simulink model "simulink_to_apollo_2015a_v2"  (R2015a)
settings: Solver=ode45  SolverMode=SingleTasking  StartTime=0.0  StopTime=inf  RelTol=1e-3
model workspace (MAT data in the model file):
  SL_ROS_VariableLengthArrays_MaxSizes.CommonInfo.ArrayTruncateAction = 'EmitWarning'
  SL_ROS_VariableLengthArrays_MaxSizes.MsgTypeMap = containers.Map
  SL_ROS_VariableLengthArrays_MaxSizes.MsgTypeMap.serialization.keys = {'my_msgs/ContiRadar', 'my_msgs/Header', 'my_msgs/RoutingRequest', 'sensor_msgs/PointCloud2'}
  SL_ROS_VariableLengthArrays_MaxSizes.MsgTypeMap.serialization.values{1}.PropertyName = 'Contiobs'
  SL_ROS_VariableLengthArrays_MaxSizes.MsgTypeMap.serialization.values{1}.DataType = 'my_msgs/ContiRadarObs'
  SL_ROS_VariableLengthArrays_MaxSizes.MsgTypeMap.serialization.values{1}.MaxLength = 9
  SL_ROS_VariableLengthArrays_MaxSizes.MsgTypeMap.serialization.values{2}.PropertyName = 'ModuleName'
  SL_ROS_VariableLengthArrays_MaxSizes.MsgTypeMap.serialization.values{2}.DataType = 'uint8'
  SL_ROS_VariableLengthArrays_MaxSizes.MsgTypeMap.serialization.values{2}.MaxLength = 1
  SL_ROS_VariableLengthArrays_MaxSizes.MsgTypeMap.serialization.values{3}(1).PropertyName = 'BlacklistedRoad'
  SL_ROS_VariableLengthArrays_MaxSizes.MsgTypeMap.serialization.values{3}(1).DataType = 'std_msgs/String'
  SL_ROS_VariableLengthArrays_MaxSizes.MsgTypeMap.serialization.values{3}(1).MaxLength = 16
  SL_ROS_VariableLengthArrays_MaxSizes.MsgTypeMap.serialization.values{3}(2).PropertyName = 'Waypoint'
  SL_ROS_VariableLengthArrays_MaxSizes.MsgTypeMap.serialization.values{3}(2).DataType = 'my_msgs/LaneWayPoint'
  SL_ROS_VariableLengthArrays_MaxSizes.MsgTypeMap.serialization.values{3}(2).MaxLength = 2
  SL_ROS_VariableLengthArrays_MaxSizes.MsgTypeMap.serialization.values{4}(1).PropertyName = 'Data'
  SL_ROS_VariableLengthArrays_MaxSizes.MsgTypeMap.serialization.values{4}(1).DataType = 'uint8'
  SL_ROS_VariableLengthArrays_MaxSizes.MsgTypeMap.serialization.values{4}(1).MaxLength = 128
  SL_ROS_VariableLengthArrays_MaxSizes.MsgTypeMap.serialization.values{4}(2).PropertyName = 'Fields'
  SL_ROS_VariableLengthArrays_MaxSizes.MsgTypeMap.serialization.values{4}(2).DataType = 'sensor_msgs/PointField'
  SL_ROS_VariableLengthArrays_MaxSizes.MsgTypeMap.serialization.values{4}(2).MaxLength = 4
  SL_ROS_VariableLengthArrays_MaxSizes.MsgTypeMap.serialization.uniformity = 0
  SL_ROS_VariableLengthArrays_MaxSizes.MsgTypeMap.serialization.keyType = 'char'
  SL_ROS_VariableLengthArrays_MaxSizes.MsgTypeMap.serialization.valueType = 'any'
undefined symbols (not defined in the file): CameraTimestamp, Confidence, ConfidenceType, Contiobs, Contiobs_SL_Info, Count, Data, Datatype, ErrorCode, Fields, Fields_SL_Info, Header, Height, Id, Id_SL_Info, Imu, Length, LidarTimestamp, Name, Name_SL_Info, ObjectListStatus, Offset, PerceptionObstacle, PerceptionObstacle_SL_Info, PointStep, PolygonPoint, PolygonPoint_SL_Info, Pose, Position, RadarTimestamp, RowStep, S, SequenceNum, Theta, Timestamp, TimestampSec, TrackingTime, Type, Velocity, Waypoint, Width, X, Y, Z
libraries: robotlib x35
settings Model: CovMetricSettings=dwe  CovHtmlReporting=off  covSaveCumulativeToWorkspaceVar=off  CovSaveSingleToWorkspaceVar=off  CovExternalEMLEnable=on  Creator=mskim  LastModifiedBy=mskim
settings DataIOCC: LimitDataPoints=off  SaveFormat=Dataset
settings DebuggingCC: SFUnexpectedBacktrackingDiag=error  SFNoUnconditionalDefaultTransitionDiag=error
settings HardwareCC: ProdBitPerPointer=64  ProdLargestAtomicFloat=Float  ProdIntDivRoundTo=Zero  ProdEndianess=LittleEndian  ProdHWDeviceType=Specified
settings ModelReferenceCC: PropagateSignalLabelsOutOfModel=on
settings SFSimCC: SimUseLocalCustomCode=on
settings RTWCC: RTWUseLocalCustomCode=on
settings GRTTargetCC: TargetLangStandard=C99 (ISO)  GeneratePreprocessorConditionals=Use local settings

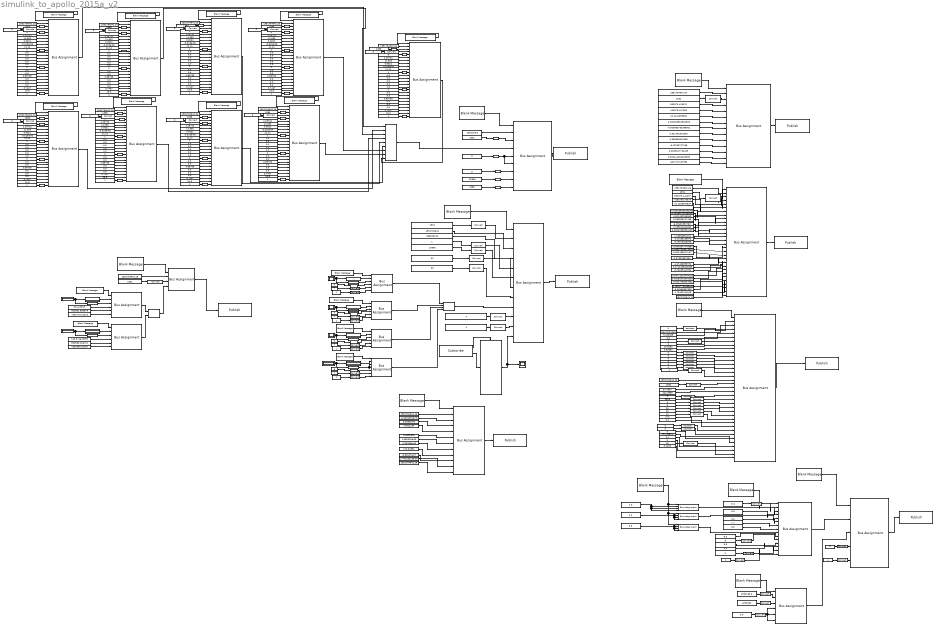
== system simulink_to_apollo_2015a_v2 ==
  note: 32
  note: 6
  note: 30
  note: 0
  note: 26
  note: 24
  note: 17
  note: 11
  Blank Message : robotlib/Blank Message  messageClass=Message  entityType=my_msgs/Gps  messageType=my_msgs/Gps  SampleTime=inf
  Blank Message1 : robotlib/Blank Message  messageClass=Message  entityType=my_msgs/LocalizationEstimate  messageType=my_msgs/LocalizationEstimate  SampleTime=inf
  Blank Message{10..18} (9 alike) : robotlib/Blank Message  messageClass=Message  entityType=my_msgs/ContiRadarObs  messageType=my_msgs/ContiRadarObs  SampleTime=inf
  Blank Message19 : robotlib/Blank Message  messageClass=Message  entityType=my_msgs/RoutingRequest  messageType=my_msgs/RoutingRequest  SampleTime=inf
  Blank Message2 : robotlib/Blank Message  messageClass=Message  entityType=my_msgs/CorrectedImu  messageType=my_msgs/CorrectedImu  SampleTime=inf
  Blank Message20 : robotlib/Blank Message  messageClass=Message  entityType=my_msgs/LaneWayPoint  messageType=my_msgs/LaneWayPoint  SampleTime=inf
  Blank Message21 : robotlib/Blank Message  messageClass=Message  entityType=my_msgs/LaneWayPoint  messageType=my_msgs/LaneWayPoint  SampleTime=inf
  Blank Message22 : robotlib/Blank Message  messageClass=Message  entityType=my_msgs/Header  messageType=my_msgs/Header  SampleTime=inf
  Blank Message23 : robotlib/Blank Message  messageClass=Message  entityType=my_msgs/PerceptionObstacle  messageType=my_msgs/PerceptionObstacle  SampleTime=inf
  Blank Message24 : robotlib/Blank Message  messageClass=Message  entityType=my_msgs/Point3D  messageType=my_msgs/Point3D  SampleTime=inf
  Blank Message25 : robotlib/Blank Message  messageClass=Message  entityType=my_msgs/PerceptionObstacles  messageType=my_msgs/PerceptionObstacles  SampleTime=inf
  Blank Message3 : robotlib/Blank Message  messageClass=Message  entityType=sensor_msgs/PointCloud2  messageType=sensor_msgs/PointCloud2  SampleTime=inf
  Blank Message{4..6,8} (4 alike) : robotlib/Blank Message  messageClass=Message  entityType=sensor_msgs/PointField  messageType=sensor_msgs/PointField  SampleTime=inf
  Blank Message7 : robotlib/Blank Message  messageClass=Message  entityType=my_msgs/Chassis  messageType=my_msgs/Chassis  SampleTime=inf
  Blank Message9 : robotlib/Blank Message  messageClass=Message  entityType=my_msgs/ContiRadar  messageType=my_msgs/ContiRadar  SampleTime=inf
  Bus Assignment : BusAssignment  AssignedSignals=Header.TimestampSec,Header.SequenceNum,Localization.Position.X,Localization.Position.Y,Localization.Position.Z,Localization.Orientation.Qx,Localization.Orientation.Qy,Localization.Orientation.Qz,Localization.Orientation.Qw,Localization.LinearVelocity.X,Localization.LinearVelocity.Y,Localization.LinearVelocity.Z,Localization.Heading
  Bus Assignment1 : BusAssignment  AssignedSignals=Header.TimestampSec,Header.SequenceNum,Pose.Position.X,Pose.Position.Y,Pose.Position.Z,Pose.Orientation.Qx,Pose.Orientation.Qy,Pose.Orientation.Qz,Pose.Orientation.Qw,Pose.LinearVelocity.X,Pose.LinearVelocity.Y,Pose.LinearVelocity.Z,Pose.LinearAccelration.X,Pose.LinearAccelration.Y,Pose.LinearAccelration.Z,Pose.AngularVelocity.X,Pose.AngularVelocity.Y,Pose.AngularVelocity.Z,Pose.Heading,Pose.LinearAccelerationVrf.X,Pose.LinearAccelerationVrf.Y,Pose.LinearAccelerationVrf.Z,Pose.AngularAccelerationVrf.X,Pose.AngularAccelerationVrf.Y,Pose.AngularAccelerationVrf.Z,Pose.EulerAngles.X,Pose.EulerAngles.Y,Pose.EulerAngles.Z,MeasurementTime
  Bus Assignment{10..18} (9 alike) : BusAssignment  AssignedSignals=Header.TimestampSec,Header.SequenceNum,Clusterortrack,ObstacleId,LongitudeDist,LateralDist,LongitudeVel,LateralVel,Rcs,Dynprop,LongitudeDistRms,LateralDistRms,LongitudeVelRms,LateralVelRms,Probexist,MeasState,LongitudeAccel,LateralAccel,OritationAngle,LongitudeAccelRms,LateralAccelRms,OritationAngleRms,Length,Width,ObstacleClass
  Bus Assignment19 : BusAssignment  AssignedSignals=Header.TimestampSec,Header.SequenceNum,Waypoint
  Bus Assignment2 : BusAssignment  AssignedSignals=Header.TimestampSec,Imu.LinearAccelration.X,Imu.LinearAccelration.Y,Imu.LinearAccelration.Z,Imu.AngularVelocity.X,Imu.AngularVelocity.Y,Imu.AngularVelocity.Z,Imu.Heading,Imu.EulerAngles.X,Imu.EulerAngles.Y,Imu.EulerAngles.Z
  Bus Assignment20 : BusAssignment  AssignedSignals=Id,Id_SL_Info.CurrentLength,S,Pose.X,Pose.Y
  Bus Assignment21 : BusAssignment  AssignedSignals=Id,Id_SL_Info.CurrentLength,S,Pose.X,Pose.Y
  Bus Assignment22 : BusAssignment  AssignedSignals=TimestampSec,SequenceNum,LidarTimestamp,CameraTimestamp,RadarTimestamp
  Bus Assignment23 : BusAssignment  AssignedSignals=Id,Position,Theta,Velocity,Length,Width,Height,PolygonPoint,TrackingTime,Type,Timestamp,Confidence,ConfidenceType,PolygonPoint_SL_Info.CurrentLength
  Bus Assignment24 : BusAssignment  AssignedSignals=X,Y,Z
  Bus Assignment25 : BusAssignment  AssignedSignals=X,Y,Z
  Bus Assignment26 : BusAssignment  AssignedSignals=X,Y,Z
  Bus Assignment27 : BusAssignment  AssignedSignals=PerceptionObstacle,Header,ErrorCode,PerceptionObstacle_SL_Info.CurrentLength
  Bus Assignment3 : BusAssignment  AssignedSignals=Header.Seq,Header.Stamp.Sec,Header.Stamp.Nsec,Height,Width,PointStep,RowStep,Fields,Fields_SL_Info.CurrentLength,Fields_SL_Info.ReceivedLength,Data
  Bus Assignment4 : BusAssignment  AssignedSignals=Name,Name_SL_Info.CurrentLength,Offset,Datatype,Count
  Bus Assignment5 : BusAssignment  AssignedSignals=Name,Name_SL_Info.CurrentLength,Offset,Datatype,Count
  Bus Assignment6 : BusAssignment  AssignedSignals=Name,Name_SL_Info.CurrentLength,Offset,Datatype,Count
  Bus Assignment7 : BusAssignment  AssignedSignals=EngineStarted,EngineRpm,SpeedMps,OdometerM,FuelRangeM,ThrottlePercentage,BrakePercentage,SteeringPercentage,ParkingBrake,HighBeamSignal,LowBeamSignal,LeftTurnSignal,RightTurnSignal,Wiper,DrivingMode,Header.TimestampSec,Header.SequenceNum,ChassisGps.Latitude,ChassisGps.Longitude,ChassisGps.GpsValid,ChassisGps.Year,ChassisGps.Month,ChassisGps.Day,ChassisGps.Hours,ChassisGps.Minutes,ChassisGps.Seconds,ChassisGps.CompassDirection,ChassisGps.Pdop,ChassisGps.IsGpsFault,ChassisGps.IsInferred,ChassisGps.Altitude,ChassisGps.Heading,ChassisGps.Hdop,ChassisGps.Vdop,ChassisGps.NumSatellites,ChassisGps.GpsSpeed
  Bus Assignment8 : BusAssignment  AssignedSignals=Name,Name_SL_Info.CurrentLength,Name_SL_Info.ReceivedLength,Offset,Datatype,Count
  Bus Assignment9 : BusAssignment  AssignedSignals=Header.TimestampSec,Header.SequenceNum,Contiobs,Contiobs_SL_Info.CurrentLength,Contiobs_SL_Info.ReceivedLength,ObjectListStatus.NofObjects,ObjectListStatus.MeasCounter,ObjectListStatus.InterfaceVersion
  Cast To Boolean{,1..9} (10 alike) : DataTypeConversion  OutDataTypeStr=boolean
  Constant{,13,81,99,110,116,141,166,191,216,241,266,291,316,341} (15 alike) : Constant  Value=1551784842.26
  Constant{1,14,44,82,111,342} (6 alike) : Constant  Value=1531
  Constant10 : Constant  Value=0.0829047784209
  Constant100 : Constant  Value=-0.0001554879
  Constant101 : Constant  Value=9.3063e-05
  Constant102 : Constant  Value=-9.811154
  Constant103 : Constant  Value=0.0001616
  Constant104 : Constant  Value=2.995926e-06
  Constant105 : Constant  Value=-2.82969e-09
  Constant106 : Constant  Value=270.84991
  Constant107 : Constant  Value=1532165.6
  Constant108 : Constant  Value=-5.81627e-07
  Constant109 : Constant  Value=2.44229215e-05
  Constant11 : Constant  Value=0.000244081020355
  Constant112 : Constant  Value=9
  Constant113 : Constant  Value=9
  Constant114 : Constant  Value=22800
  Constant115 : Constant  Value=1386
  Constant{117,142,167,192,217,242,267,292,317} (9 alike) : Constant  Value=1385
  Constant{118,143,168,193,218,243,268,293,318} (9 alike) : Constant  Value=2.25722
  Constant{42..43,45..46,55..57,63,70..71,91..92,98,119,144,169,194,219,244,269..270,294,319,352} (24 alike) : Constant  Value=0
  Constant12 : Constant  Value=-225.727157593
  Constant120 : Constant  Value=6
  Constant{121,146,171,196,221,246,271,296,321} (9 alike) : Constant  Value=11.933
  Constant{122,147,172,197,222,247,272,297,322} (9 alike) : Constant  Value=-3.619e-06
  Constant{123,148,173,198,223,248,273,298,323} (9 alike) : Constant  Value=0.0021
  Constant{124,149,174,199,224,249,274,299,324} (9 alike) : Constant  Value=11.11
  Constant{69,125,127..129,131,133..134,136,138,150,152..154,156,158..159,161,163,175,177..179,181,183..184,186,188,200,202..204,206,208..209,211,213,225,227..229,231,233..234,236,238,250,252..254,256,258..259,261,263,275,277..279,281,283..284,286,288,300,302..304,306,308..309,311,313,325,327..329,331,333..334,336,338,361} (83 alike) : Constant  Value=0.0
  Constant{49,53,65..66,76,79..80,126,140,151,165,176,190,201,215,226,240,251,265,276,290,295,301,315,326,340,357..359} (29 alike) : Constant
  Constant{130,155,180,205,230,255,280,305,330,364} (10 alike) : Constant  Value=1.0
  Constant{95,132,157,182,207,220,232,257,282,307,332} (11 alike) : Constant  Value=2
  Constant{135,160,185,210,235,260,285,310,335} (9 alike) : Constant  Value=0.85705
  Constant{137,162,187,212,237,262,287,312,337} (9 alike) : Constant  Value=3.7407
  Constant{139,164,189,214,239,264,289,314,339} (9 alike) : Constant  Value=10.6
  Constant{52,62,64,75,145} (5 alike) : Constant  Value=7
  Constant15 : Constant  Value=0.00012568384409
  Constant16 : Constant  Value=1.10996984434
  Constant17 : Constant  Value=-1.27253139942
  Constant{51,59..60,170} (4 alike) : Constant  Value=4
  Constant18 : Constant  Value=552873.141037
  Constant19 : Constant  Value=4182766.70679
  Constant195 : Constant  Value=5
  Constant2 : Constant  Value=552870.429222
  Constant20 : Constant  Value=10.1238040924
  Constant21 : Constant  Value=0.000253551552305
  Constant22 : Constant  Value=-0.000893782998901
  Constant23 : Constant  Value=0.921432316303
  Constant24 : Constant  Value=-6.19401931763
  Constant245 : Constant  Value=3
  Constant25 : Constant  Value=0.139211624861
  Constant26 : Constant  Value=-9.75978325506
  Constant27 : Constant  Value=-0.0043677779987
  Constant28 : Constant  Value=0.00567089976961
  Constant29 : Constant  Value=-0.0024595711077
  Constant3 : Constant  Value=4182784.07053
  Constant30 : Constant  Value=-2.37322587092
  Constant31 : Constant  Value=-1.67436599731
  Constant32 : Constant  Value=0.0740453600883
  Constant320 : Constant  Value=8
  Constant33 : Constant  Value=0.390536427498
  Constant34 : Constant  Value=-9.76195441931
  Constant343 : Constant  Value=20.412915
  Constant344 : Constant  Value=552881.650878
  Constant345 : Constant  Value=4182775.01019
  Constant346 : Constant  Value=113.374625055
  Constant347 : Constant  Value=552880.126721
  Constant348 : Constant  Value=4182806.92204
  Constant349 : Constant  Value=1532165.6
  Constant35 : Constant  Value=0.00711610494182
  Constant350 : Constant  Value=3.5
  Constant351 : Constant  Value=111
  Constant353 : Constant  Value=9.9
  Constant354 : Constant  Value=6.6
  Constant355 : Constant  Value=5
  Constant356 : Constant  Value=8.8
  Constant36 : Constant  Value=-0.000803495408036
  Constant360 : Constant  Value=4092962
  Constant362 : Constant  Value=2.2
  Constant363 : Constant  Value=5.5
  Constant365 : Constant  Value=6.6
  Constant366 : Constant  Value=7.7
  Constant367 : Constant  Value=8.8
  Constant37 : Constant  Value=-0.0024498004932
  Constant38 : Constant  Value=2.16947784683e-05
  Constant39 : Constant  Value=-6.28168967593
  Constant4 : Constant  Value=10.1241359982
  Constant40 : Constant  Value=4.73462104918
  Constant41 : Constant  Value=1551784841.11
  Constant47 : Constant  Value=1551784842
  Constant48 : Constant  Value=696618240
  Constant5 : Constant  Value=0.000253551552305
  Constant50 : Constant  Value=10966
  Constant54 : Constant  Value=32
  Constant58 : Constant  Value=99
  Constant6 : Constant  Value=-0.000893782998901
  Constant61 : Constant  Value=8
  Constant67 : Constant  Value=2536.82299805
  Constant68 : Constant  Value=5.123308
  Constant7 : Constant  Value=0.921432316303
  Constant72 : Constant  Value=18.5281
  Constant73 : Constant  Value=0.69582
  Constant74 : Constant  Value=8
  Constant77 : Constant  Value=37.7907
  Constant78 : Constant  Value=-122.3995
  Constant8 : Constant  Value=0.388538002968
  Constant83 : Constant  Value=2019
  Constant84 : Constant  Value=3
  Constant85 : Constant  Value=5
  Constant86 : Constant  Value=20
  Constant87 : Constant  Value=20
  Constant88 : Constant  Value=41
  Constant89 : Constant  Value=270
  Constant9 : Constant  Value=-5.12263727188
  Constant90 : Constant  Value=0.1
  Constant93 : Constant  Value=271.02511
  Constant94 : Constant  Value=0.1
  Constant96 : Constant  Value=15
  Constant97 : Constant  Value=5.1233
  Data Type Conversion{,1..99} (100 alike) : DataTypeConversion
  Enabled Subsystem : Subsystem
  Matrix Concatenate : Concatenate  NumInputs=4  Mode=Multidimensional array  ConcatenateDimension=2
  Matrix Concatenate1 : Concatenate  NumInputs=9  Mode=Multidimensional array  ConcatenateDimension=2
  Matrix Concatenate2 : Concatenate  Mode=Multidimensional array  ConcatenateDimension=2
  Publish1 : robotlib/Publish  topicSource=Specify your own  topic=/my_msgs/Gps  messageType=my_msgs/Gps  messageQueueLength=1
  Publish2 : robotlib/Publish  topicSource=Specify your own  topic=/my_msgs/LocalizationEstimate  messageType=my_msgs/LocalizationEstimate  messageQueueLength=1
  Publish3 : robotlib/Publish  topicSource=Specify your own  topic=/my_msgs/CorrectedImu  messageType=my_msgs/CorrectedImu  messageQueueLength=1
  Publish4 : robotlib/Publish  topicSource=Specify your own  topic=/sensor_msgs/PointCloud2  messageType=sensor_msgs/PointCloud2  messageQueueLength=1
  Publish5 : robotlib/Publish  topicSource=Specify your own  topic=/my_msgs/Chassis  messageType=my_msgs/Chassis  messageQueueLength=1
  Publish6 : robotlib/Publish  topicSource=Specify your own  topic=/my_msgs/ContiRadar  messageType=my_msgs/ContiRadar  messageQueueLength=1
  Publish7 : robotlib/Publish  topicSource=Specify your own  topic=/my_msgs/RoutingRequest  messageType=my_msgs/RoutingRequest  messageQueueLength=1
  Publish8 : robotlib/Publish  topicSource=Specify your own  topic=/my_msgs/PerceptionObstacles  messageType=my_msgs/PerceptionObstacles  messageQueueLength=1
  Scope : Scope
      settings: TimeRange=auto  MaxDataPoints=5000  SaveToWorkspace=off  SaveName=ScopeData  YMin=-31.875  YMax=286.875  SampleTime=-1
  String Constant1 : Subsystem  Description=Replaced Block  mask(Replaced Block){}
      mask help: This block has been replaced with an empty subsystem because it used functionality that is unavailable in Simulink R2015a.
      mask Display: fprintf('Replaced: %s\n','StringConstant')
  String Constant2 : Subsystem  Description=Replaced Block  mask(Replaced Block){}
      mask help: This block has been replaced with an empty subsystem because it used functionality that is unavailable in Simulink R2015a.
      mask Display: fprintf('Replaced: %s\n','StringConstant')
  String Constant3 : Subsystem  Description=Replaced Block  mask(Replaced Block){}
      mask help: This block has been replaced with an empty subsystem because it used functionality that is unavailable in Simulink R2015a.
      mask Display: fprintf('Replaced: %s\n','StringConstant')
  String Constant4 : Subsystem  Description=Replaced Block  mask(Replaced Block){}
      mask help: This block has been replaced with an empty subsystem because it used functionality that is unavailable in Simulink R2015a.
      mask Display: fprintf('Replaced: %s\n','StringConstant')
  String Constant5 : Subsystem  Description=Replaced Block  mask(Replaced Block){}
      mask help: This block has been replaced with an empty subsystem because it used functionality that is unavailable in Simulink R2015a.
      mask Display: fprintf('Replaced: %s\n','StringConstant')
  String Constant6 : Subsystem  Description=Replaced Block  mask(Replaced Block){}
      mask help: This block has been replaced with an empty subsystem because it used functionality that is unavailable in Simulink R2015a.
      mask Display: fprintf('Replaced: %s\n','StringConstant')
  String Length1 : Subsystem  Description=Replaced Block  mask(Replaced Block){}
      mask help: This block has been replaced with an empty subsystem because it used functionality that is unavailable in Simulink R2015a.
      mask Display: fprintf('Replaced: %s\n','StringLength')
  String Length2 : Subsystem  Description=Replaced Block  mask(Replaced Block){}
      mask help: This block has been replaced with an empty subsystem because it used functionality that is unavailable in Simulink R2015a.
      mask Display: fprintf('Replaced: %s\n','StringLength')
  String Length3 : Subsystem  Description=Replaced Block  mask(Replaced Block){}
      mask help: This block has been replaced with an empty subsystem because it used functionality that is unavailable in Simulink R2015a.
      mask Display: fprintf('Replaced: %s\n','StringLength')
  String Length4 : Subsystem  Description=Replaced Block  mask(Replaced Block){}
      mask help: This block has been replaced with an empty subsystem because it used functionality that is unavailable in Simulink R2015a.
      mask Display: fprintf('Replaced: %s\n','StringLength')
  String Length5 : Subsystem  Description=Replaced Block  mask(Replaced Block){}
      mask help: This block has been replaced with an empty subsystem because it used functionality that is unavailable in Simulink R2015a.
      mask Display: fprintf('Replaced: %s\n','StringLength')
  String Length6 : Subsystem  Description=Replaced Block  mask(Replaced Block){}
      mask help: This block has been replaced with an empty subsystem because it used functionality that is unavailable in Simulink R2015a.
      mask Display: fprintf('Replaced: %s\n','StringLength')
  String to ASCII1 : Subsystem  Description=Replaced Block  mask(Replaced Block){}
      mask help: This block has been replaced with an empty subsystem because it used functionality that is unavailable in Simulink R2015a.
      mask Display: fprintf('Replaced: %s\n','StringToASCII')
  String to ASCII2 : Subsystem  Description=Replaced Block  mask(Replaced Block){}
      mask help: This block has been replaced with an empty subsystem because it used functionality that is unavailable in Simulink R2015a.
      mask Display: fprintf('Replaced: %s\n','StringToASCII')
  String to ASCII3 : Subsystem  Description=Replaced Block  mask(Replaced Block){}
      mask help: This block has been replaced with an empty subsystem because it used functionality that is unavailable in Simulink R2015a.
      mask Display: fprintf('Replaced: %s\n','StringToASCII')
  String to ASCII4 : Subsystem  Description=Replaced Block  mask(Replaced Block){}
      mask help: This block has been replaced with an empty subsystem because it used functionality that is unavailable in Simulink R2015a.
      mask Display: fprintf('Replaced: %s\n','StringToASCII')
  String to ASCII5 : Subsystem  Description=Replaced Block  mask(Replaced Block){}
      mask help: This block has been replaced with an empty subsystem because it used functionality that is unavailable in Simulink R2015a.
      mask Display: fprintf('Replaced: %s\n','StringToASCII')
  String to ASCII6 : Subsystem  Description=Replaced Block  mask(Replaced Block){}
      mask help: This block has been replaced with an empty subsystem because it used functionality that is unavailable in Simulink R2015a.
      mask Display: fprintf('Replaced: %s\n','StringToASCII')
  Subscribe1 : robotlib/Subscribe  topicSource=Specify your own  topic=/apollo/sensor/velodyne64/compensator/PointCloud2  messageType=sensor_msgs/PointCloud2  sampleTime=-1  messageQueueLength=51
  wires:
  Constant4/1 -> Bus Assignment/6
  Data Type Conversion/1 -> Bus Assignment/3
  Constant6/1 -> Bus Assignment/8
  Constant12/1 -> Bus Assignment/14
  Constant9/1 -> Bus Assignment/11
  Constant5/1 -> Bus Assignment/7
  Constant7/1 -> Bus Assignment/9
  Constant1/1 -> Data Type Conversion/1
  Constant2/1 -> Bus Assignment/4
  Constant3/1 -> Bus Assignment/5
  Blank Message/1 -> Bus Assignment/1
  Bus Assignment/1 -> Publish1/1
  Constant8/1 -> Bus Assignment/10
  Constant11/1 -> Bus Assignment/13
  Constant10/1 -> Bus Assignment/12
  Constant/1 -> Bus Assignment/2
  Constant13/1 -> Bus Assignment1/2
  Constant18/1 -> Bus Assignment1/4
  Constant19/1 -> Bus Assignment1/5
  Constant21/1 -> Bus Assignment1/7
  Bus Assignment1/1 -> Publish2/1
  Blank Message1/1 -> Bus Assignment1/1
  Constant14/1 -> Data Type Conversion1/1
  Data Type Conversion1/1 -> Bus Assignment1/3
  Constant20/1 -> Bus Assignment1/6
  Constant22/1 -> Bus Assignment1/8
  Constant23/1 -> Bus Assignment1/9
  Constant33/1 -> Bus Assignment1/10
  Constant24/1 -> Bus Assignment1/11
  Constant25/1 -> Bus Assignment1/12
  Constant15/1 -> Bus Assignment1/13
  Constant16/1 -> Bus Assignment1/14
  Constant17/1 -> Bus Assignment1/15
  Constant26/1 -> Bus Assignment1/16
  Constant27/1 -> Bus Assignment1/17
  Constant28/1 -> Bus Assignment1/18
  Constant29/1 -> Bus Assignment1/19
  Constant30/1 -> Bus Assignment1/20
  Constant31/1 -> Bus Assignment1/21
  Constant32/1 -> Bus Assignment1/22
  Constant34/1 -> Bus Assignment1/23
  Constant35/1 -> Bus Assignment1/24
  Constant36/1 -> Bus Assignment1/25
  Constant37/1 -> Bus Assignment1/26
  Constant38/1 -> Bus Assignment1/27
  Constant39/1 -> Bus Assignment1/28
  Constant40/1 -> Bus Assignment1/29
  Constant41/1 -> Bus Assignment1/30
  Blank Message3/1 -> Bus Assignment3/1
  Constant50/1 -> Data Type Conversion6/1
  Bus Assignment3/1 -> Publish4/1
  String Length3/1(Out1) -> Bus Assignment4/3
  Data Type Conversion8/1 -> Bus Assignment3/8
  Data Type Conversion7/1 -> Bus Assignment3/7
  Constant54/1 -> Data Type Conversion7/1
  Data Type Conversion6/1 -> Bus Assignment3/6
  Constant64/1 -> Data Type Conversion10/1
  Data Type Conversion5/1 -> Bus Assignment3/5
  Constant47/1 -> Bus Assignment3/3
  Data Type Conversion11/1 -> Bus Assignment4/6
  Data Type Conversion9/1 -> Bus Assignment4/4
  Constant63/1 -> Data Type Conversion9/1
  Blank Message4/1 -> Bus Assignment4/1
  Data Type Conversion10/1 -> Bus Assignment4/5
  String Constant3/1(Out1) -> String Length3/1(In1), String to ASCII1/1(In1)
  String to ASCII1/1(Out1) -> Bus Assignment4/2
  Constant58/1 -> Data Type Conversion8/1
  Constant44/1 -> Data Type Conversion4/1
  Constant48/1 -> Bus Assignment3/4
  Constant49/1 -> Data Type Conversion5/1
  Data Type Conversion4/1 -> Bus Assignment3/2
  Constant65/1 -> Data Type Conversion11/1
  Bus Assignment4/1 -> Matrix Concatenate/1
  Constant59/1 -> Data Type Conversion15/1
  Constant60/1 -> Data Type Conversion16/1
  Constant53/1 -> Data Type Conversion13/1
  String Constant1/1(Out1) -> String Length1/1(In1), String to ASCII2/1(In1)
  Data Type Conversion14/1 -> Bus Assignment5/4
  Constant52/1 -> Data Type Conversion12/1
  Data Type Conversion13/1 -> Bus Assignment5/6
  String Length1/1(Out1) -> Bus Assignment5/3
  String to ASCII2/1(Out1) -> Bus Assignment5/2
  Blank Message5/1 -> Bus Assignment5/1
  Constant51/1 -> Data Type Conversion14/1
  Data Type Conversion12/1 -> Bus Assignment5/5
  Constant66/1 -> Data Type Conversion18/1
  String Constant2/1(Out1) -> String Length2/1(In1), String to ASCII3/1(In1)
  Data Type Conversion19/1 -> Bus Assignment6/4
  Constant62/1 -> Data Type Conversion17/1
  Data Type Conversion18/1 -> Bus Assignment6/6
  String Length2/1(Out1) -> Bus Assignment6/3
  String to ASCII3/1(Out1) -> Bus Assignment6/2
  Blank Message6/1 -> Bus Assignment6/1
  Constant61/1 -> Data Type Conversion19/1
  Data Type Conversion17/1 -> Bus Assignment6/5
  Matrix Concatenate/1 -> Bus Assignment3/9
  Data Type Conversion15/1 -> Bus Assignment3/10
  Data Type Conversion16/1 -> Bus Assignment3/11
  Bus Assignment5/1 -> Matrix Concatenate/2
  Bus Assignment6/1 -> Matrix Concatenate/3
  Constant76/1 -> Data Type Conversion26/1
  Bus Assignment8/1 -> Matrix Concatenate/4
  String to ASCII4/1(Out1) -> Bus Assignment8/2
  Constant74/1 -> Data Type Conversion27/1
  String Constant4/1(Out1) -> String Length4/1(In1), String to ASCII4/1(In1)
  Blank Message8/1 -> Bus Assignment8/1
  String Length4/1(Out1) -> Bus Assignment8/4, Bus Assignment8/3
  Constant75/1 -> Data Type Conversion25/1
  Data Type Conversion27/1 -> Bus Assignment8/5
  Data Type Conversion25/1 -> Bus Assignment8/6
  Data Type Conversion26/1 -> Bus Assignment8/7
  Blank Message7/1 -> Bus Assignment7/1
  Bus Assignment7/1 -> Publish5/1
  Constant42/1 -> Cast To Boolean/1
  Cast To Boolean/1 -> Bus Assignment7/2
  Constant67/1 -> Bus Assignment7/3
  Constant68/1 -> Bus Assignment7/4
  Constant69/1 -> Bus Assignment7/5
  Constant70/1 -> Data Type Conversion2/1
  Constant71/1 -> Bus Assignment7/7
  Constant43/1 -> Cast To Boolean1/1
  Constant45/1 -> Cast To Boolean2/1
  Constant46/1 -> Cast To Boolean3/1
  Constant57/1 -> Cast To Boolean6/1
  Constant56/1 -> Cast To Boolean5/1
  Constant55/1 -> Cast To Boolean4/1
  Constant72/1 -> Bus Assignment7/8
  Constant73/1 -> Bus Assignment7/9
  Cast To Boolean1/1 -> Bus Assignment7/10
  Cast To Boolean2/1 -> Bus Assignment7/11
  Cast To Boolean3/1 -> Bus Assignment7/12
  Cast To Boolean4/1 -> Bus Assignment7/13
  Cast To Boolean5/1 -> Bus Assignment7/14
  Cast To Boolean6/1 -> Bus Assignment7/15
  Constant80/1 -> Data Type Conversion3/1
  Constant82/1 -> Data Type Conversion20/1
  Constant81/1 -> Bus Assignment7/17
  Constant79/1 -> Cast To Boolean7/1
  Constant91/1 -> Cast To Boolean8/1
  Constant98/1 -> Cast To Boolean9/1
  Constant83/1 -> Data Type Conversion21/1
  Constant84/1 -> Data Type Conversion22/1
  Constant85/1 -> Data Type Conversion23/1
  Constant86/1 -> Data Type Conversion24/1
  Constant87/1 -> Data Type Conversion28/1
  Constant88/1 -> Data Type Conversion29/1
  Constant96/1 -> Data Type Conversion30/1
  Data Type Conversion2/1 -> Bus Assignment7/6
  Data Type Conversion3/1 -> Bus Assignment7/16
  Data Type Conversion20/1 -> Bus Assignment7/18
  Constant77/1 -> Bus Assignment7/19
  Constant78/1 -> Bus Assignment7/20
  Cast To Boolean7/1 -> Bus Assignment7/21
  Data Type Conversion21/1 -> Bus Assignment7/22
  Data Type Conversion22/1 -> Bus Assignment7/23
  Data Type Conversion23/1 -> Bus Assignment7/24
  Data Type Conversion24/1 -> Bus Assignment7/25
  Data Type Conversion28/1 -> Bus Assignment7/26
  Data Type Conversion29/1 -> Bus Assignment7/27
  Constant89/1 -> Bus Assignment7/28
  Constant90/1 -> Bus Assignment7/29
  Cast To Boolean8/1 -> Bus Assignment7/30
  Cast To Boolean9/1 -> Bus Assignment7/31
  Constant92/1 -> Bus Assignment7/32
  Constant93/1 -> Bus Assignment7/33
  Constant94/1 -> Bus Assignment7/34
  Constant95/1 -> Bus Assignment7/35
  Data Type Conversion30/1 -> Bus Assignment7/36
  Constant97/1 -> Bus Assignment7/37
  Blank Message2/1 -> Bus Assignment2/1
  Bus Assignment2/1 -> Publish3/1
  Constant99/1 -> Bus Assignment2/2
  Constant100/1 -> Bus Assignment2/3
  Constant101/1 -> Bus Assignment2/4
  Constant102/1 -> Bus Assignment2/5
  Constant103/1 -> Bus Assignment2/6
  Constant104/1 -> Bus Assignment2/7
  Constant105/1 -> Bus Assignment2/8
  Constant106/1 -> Bus Assignment2/9
  Constant108/1 -> Bus Assignment2/10
  Constant109/1 -> Bus Assignment2/11
  Constant110/1 -> Bus Assignment2/12
  Subscribe1/2 -> Enabled Subsystem/1(In1)
  Subscribe1/1 -> Enabled Subsystem/Enable
  Enabled Subsystem/1(Out1) -> Scope/1, Bus Assignment3/12
  Blank Message9/1 -> Bus Assignment9/1
  Bus Assignment9/1 -> Publish6/1
  Constant327/1 -> Bus Assignment18/13
  Constant316/1 -> Bus Assignment18/2
  Constant339/1 -> Bus Assignment18/25
  Constant318/1 -> Bus Assignment18/6
  Constant336/1 -> Bus Assignment18/22
  Constant322/1 -> Bus Assignment18/9
  Constant330/1 -> Bus Assignment18/16
  Constant324/1 -> Bus Assignment18/10
  Constant319/1 -> Data Type Conversion39/1
  Constant334/1 -> Bus Assignment18/21
  Constant328/1 -> Bus Assignment18/15
  Constant325/1 -> Bus Assignment18/12
  Constant323/1 -> Bus Assignment18/8
  Constant333/1 -> Bus Assignment18/19
  Constant335/1 -> Bus Assignment18/20
  Data Type Conversion39/1 -> Bus Assignment18/4
  Constant338/1 -> Bus Assignment18/23
  Constant321/1 -> Bus Assignment18/7
  Constant337/1 -> Bus Assignment18/24
  Constant329/1 -> Bus Assignment18/14
  Constant331/1 -> Bus Assignment18/18
  Blank Message18/1 -> Bus Assignment18/1
  Constant317/1 -> Data Type Conversion42/1
  Data Type Conversion42/1 -> Bus Assignment18/3
  Constant340/1 -> Data Type Conversion49/1
  Data Type Conversion49/1 -> Bus Assignment18/26
  Constant332/1 -> Data Type Conversion50/1
  Data Type Conversion50/1 -> Bus Assignment18/17
  Constant326/1 -> Data Type Conversion61/1
  Data Type Conversion61/1 -> Bus Assignment18/11
  Constant320/1 -> Data Type Conversion83/1
  Data Type Conversion83/1 -> Bus Assignment18/5
  Bus Assignment18/1 -> Matrix Concatenate1/9
  Constant107/1 -> Bus Assignment9/2
  Constant111/1 -> Data Type Conversion31/1
  Data Type Conversion31/1 -> Bus Assignment9/3
  Constant112/1 -> Data Type Conversion32/1
  Data Type Conversion32/1 -> Bus Assignment9/6, Bus Assignment9/5
  Constant113/1 -> Data Type Conversion87/1
  Constant114/1 -> Data Type Conversion88/1
  Constant115/1 -> Data Type Conversion89/1
  Bus Assignment12/1 -> Matrix Concatenate1/5
  Bus Assignment14/1 -> Matrix Concatenate1/3
  Bus Assignment15/1 -> Matrix Concatenate1/4
  Bus Assignment16/1 -> Matrix Concatenate1/1
  Bus Assignment13/1 -> Matrix Concatenate1/6
  Constant287/1 -> Bus Assignment16/24
  Blank Message13/1 -> Bus Assignment13/1
  Data Type Conversion54/1 -> Bus Assignment11/26
  Data Type Conversion47/1 -> Bus Assignment15/3
  Constant188/1 -> Bus Assignment12/23
  Constant263/1 -> Bus Assignment15/23
  Data Type Conversion70/1 -> Bus Assignment14/17
  Data Type Conversion45/1 -> Bus Assignment12/3
  Constant283/1 -> Bus Assignment16/19
  Constant190/1 -> Data Type Conversion57/1
  Data Type Conversion73/1 -> Bus Assignment17/26
  Constant241/1 -> Bus Assignment15/2
  Blank Message10/1 -> Bus Assignment10/1
  Constant289/1 -> Bus Assignment16/25
  Constant119/1 -> Data Type Conversion33/1
  Constant142/1 -> Data Type Conversion44/1
  Bus Assignment11/1 -> Matrix Concatenate1/8
  Data Type Conversion56/1 -> Bus Assignment13/17
  Blank Message12/1 -> Bus Assignment12/1
  Constant181/1 -> Bus Assignment12/18
  Constant173/1 -> Bus Assignment12/8
  Constant202/1 -> Bus Assignment13/13
  Data Type Conversion74/1 -> Bus Assignment17/17
  Constant194/1 -> Data Type Conversion36/1
  Constant245/1 -> Data Type Conversion86/1
  Blank Message14/1 -> Bus Assignment14/1
  Data Type Conversion57/1 -> Bus Assignment12/26
  Constant133/1 -> Bus Assignment10/19
  Constant199/1 -> Bus Assignment13/10
  Constant205/1 -> Bus Assignment13/16
  Constant152/1 -> Bus Assignment11/13
  Constant209/1 -> Bus Assignment13/21
  Constant295/1 -> Data Type Conversion75/1
  Constant157/1 -> Data Type Conversion53/1
  Constant162/1 -> Bus Assignment11/24
  Constant216/1 -> Bus Assignment14/2
  Constant144/1 -> Data Type Conversion34/1
  Constant186/1 -> Bus Assignment12/22
  Constant309/1 -> Bus Assignment17/21
  Constant178/1 -> Bus Assignment12/15
  Constant265/1 -> Data Type Conversion66/1
  Data Type Conversion40/1 -> Bus Assignment16/4
  Constant300/1 -> Bus Assignment17/12
  Constant184/1 -> Bus Assignment12/21
  Constant177/1 -> Bus Assignment12/13
  Constant166/1 -> Bus Assignment12/2
  Constant310/1 -> Bus Assignment17/20
  Constant260/1 -> Bus Assignment15/20
  Constant180/1 -> Bus Assignment12/16
  Constant153/1 -> Bus Assignment11/15
  Constant187/1 -> Bus Assignment12/24
  Constant228/1 -> Bus Assignment14/15
  Constant185/1 -> Bus Assignment12/20
  Constant254/1 -> Bus Assignment15/14
  Constant313/1 -> Bus Assignment17/23
  Blank Message17/1 -> Bus Assignment17/1
  Constant167/1 -> Data Type Conversion45/1
  Constant222/1 -> Bus Assignment14/9
  Constant210/1 -> Bus Assignment13/20
  Constant269/1 -> Data Type Conversion40/1
  Constant305/1 -> Bus Assignment17/16
  Constant259/1 -> Bus Assignment15/21
  Constant244/1 -> Data Type Conversion38/1
  Constant273/1 -> Bus Assignment16/8
  Constant249/1 -> Bus Assignment15/10
  Constant163/1 -> Bus Assignment11/23
  Constant179/1 -> Bus Assignment12/14
  Constant141/1 -> Bus Assignment11/2
  Constant250/1 -> Bus Assignment15/12
  Constant197/1 -> Bus Assignment13/9
  Constant294/1 -> Data Type Conversion41/1
  Constant149/1 -> Bus Assignment11/10
  Constant271/1 -> Bus Assignment16/7
  Constant164/1 -> Bus Assignment11/25
  Constant158/1 -> Bus Assignment11/19
  Constant218/1 -> Bus Assignment14/6
  Constant132/1 -> Data Type Conversion62/1
  Constant277/1 -> Bus Assignment16/13
  Constant243/1 -> Bus Assignment15/6
  Constant148/1 -> Bus Assignment11/8
  Constant279/1 -> Bus Assignment16/14
  Constant285/1 -> Bus Assignment16/20
  Constant156/1 -> Bus Assignment11/18
  Constant253/1 -> Bus Assignment15/15
  Constant308/1 -> Bus Assignment17/19
  Constant195/1 -> Data Type Conversion84/1
  Constant234/1 -> Bus Assignment14/21
  Constant137/1 -> Bus Assignment10/24
  Constant139/1 -> Bus Assignment10/25
  Constant297/1 -> Bus Assignment17/9
  Constant236/1 -> Bus Assignment14/22
  Constant125/1 -> Bus Assignment10/12
  Constant238/1 -> Bus Assignment14/23
  Constant230/1 -> Bus Assignment14/16
  Constant128/1 -> Bus Assignment10/15
  Constant219/1 -> Data Type Conversion37/1
  Constant154/1 -> Bus Assignment11/14
  Bus Assignment17/1 -> Matrix Concatenate1/2
  Constant296/1 -> Bus Assignment17/7
  Data Type Conversion44/1 -> Bus Assignment11/3
  Constant256/1 -> Bus Assignment15/18
  Constant235/1 -> Bus Assignment14/20
  Data Type Conversion41/1 -> Bus Assignment17/4
  Constant226/1 -> Data Type Conversion71/1
  Constant229/1 -> Bus Assignment14/14
  Constant246/1 -> Bus Assignment15/7
  Constant312/1 -> Bus Assignment17/24
  Constant281/1 -> Bus Assignment16/18
  Constant266/1 -> Bus Assignment16/2
  Constant159/1 -> Bus Assignment11/21
  Constant247/1 -> Bus Assignment15/9
  Constant237/1 -> Bus Assignment14/24
  Data Type Conversion85/1 -> Bus Assignment11/5
  Constant264/1 -> Bus Assignment15/25
  Constant311/1 -> Bus Assignment17/22
  Constant221/1 -> Bus Assignment14/7
  Blank Message16/1 -> Bus Assignment16/1
  Constant182/1 -> Data Type Conversion58/1
  Constant275/1 -> Bus Assignment16/12
  Data Type Conversion38/1 -> Bus Assignment15/4
  Constant136/1 -> Bus Assignment10/22
  Constant223/1 -> Bus Assignment14/8
  Constant116/1 -> Bus Assignment10/2
  Data Type Conversion43/1 -> Bus Assignment10/3
  Data Type Conversion77/1 -> Bus Assignment16/26
  Data Type Conversion58/1 -> Bus Assignment12/17
  Constant127/1 -> Bus Assignment10/13
  Constant315/1 -> Data Type Conversion73/1
  Constant261/1 -> Bus Assignment15/22
  Constant220/1 -> Data Type Conversion72/1
  Constant140/1 -> Data Type Conversion63/1
  Constant227/1 -> Bus Assignment14/13
  Data Type Conversion82/1 -> Bus Assignment12/5
  Constant165/1 -> Data Type Conversion54/1
  Constant200/1 -> Bus Assignment13/12
  Constant143/1 -> Bus Assignment11/6
  Constant176/1 -> Data Type Conversion59/1
  Data Type Conversion71/1 -> Bus Assignment14/11
  Constant175/1 -> Bus Assignment12/12
  Data Type Conversion79/1 -> Bus Assignment16/11
  Constant161/1 -> Bus Assignment11/22
  Constant198/1 -> Bus Assignment13/8
  Constant239/1 -> Bus Assignment14/25
  Constant314/1 -> Bus Assignment17/25
  Constant306/1 -> Bus Assignment17/18
  Data Type Conversion35/1 -> Bus Assignment12/4
  Constant232/1 -> Data Type Conversion70/1
  Constant257/1 -> Data Type Conversion67/1
  Constant189/1 -> Bus Assignment12/25
  Constant302/1 -> Bus Assignment17/13
  Constant124/1 -> Bus Assignment10/10
  Constant252/1 -> Bus Assignment15/13
  Data Type Conversion51/1 -> Bus Assignment17/3
  Data Type Conversion55/1 -> Bus Assignment13/26
  Data Type Conversion86/1 -> Bus Assignment15/5
  Data Type Conversion67/1 -> Bus Assignment15/17
  Data Type Conversion66/1 -> Bus Assignment15/26
  Constant301/1 -> Data Type Conversion76/1
  Constant299/1 -> Bus Assignment17/10
  Constant171/1 -> Bus Assignment12/7
  Constant270/1 -> Data Type Conversion80/1
  Constant280/1 -> Bus Assignment16/16
  Data Type Conversion60/1 -> Bus Assignment10/11
  Constant192/1 -> Data Type Conversion48/1
  Constant258/1 -> Bus Assignment15/19
  Constant172/1 -> Bus Assignment12/9
  Constant278/1 -> Bus Assignment16/15
  Constant286/1 -> Bus Assignment16/22
  Constant155/1 -> Bus Assignment11/16
  Data Type Conversion72/1 -> Bus Assignment14/5
  Blank Message11/1 -> Bus Assignment11/1
  Constant122/1 -> Bus Assignment10/9
  Constant123/1 -> Bus Assignment10/8
  Constant196/1 -> Bus Assignment13/7
  Constant134/1 -> Bus Assignment10/21
  Constant191/1 -> Bus Assignment13/2
  Data Type Conversion34/1 -> Bus Assignment11/4
  Constant292/1 -> Data Type Conversion51/1
  Data Type Conversion64/1 -> Bus Assignment11/11
  Constant282/1 -> Data Type Conversion78/1
  Data Type Conversion53/1 -> Bus Assignment11/17
  Constant248/1 -> Bus Assignment15/8
  Constant126/1 -> Data Type Conversion60/1
  Constant284/1 -> Bus Assignment16/21
  Data Type Conversion59/1 -> Bus Assignment12/11
  Constant151/1 -> Data Type Conversion64/1
  Data Type Conversion65/1 -> Bus Assignment13/11
  Constant240/1 -> Data Type Conversion69/1
  Constant129/1 -> Bus Assignment10/14
  Constant160/1 -> Bus Assignment11/20
  Constant145/1 -> Data Type Conversion85/1
  Constant193/1 -> Bus Assignment13/6
  Data Type Conversion75/1 -> Bus Assignment17/5
  Constant150/1 -> Bus Assignment11/12
  Constant121/1 -> Bus Assignment10/7
  Data Type Conversion78/1 -> Bus Assignment16/17
  Constant225/1 -> Bus Assignment14/12
  Constant170/1 -> Data Type Conversion82/1
  Constant118/1 -> Bus Assignment10/6
  Constant131/1 -> Bus Assignment10/18
  Constant203/1 -> Bus Assignment13/15
  Data Type Conversion52/1 -> Bus Assignment16/3
  Blank Message15/1 -> Bus Assignment15/1
  Constant288/1 -> Bus Assignment16/23
  Data Type Conversion63/1 -> Bus Assignment10/26
  Data Type Conversion84/1 -> Bus Assignment13/5
  Constant303/1 -> Bus Assignment17/15
  Data Type Conversion68/1 -> Bus Assignment15/11
  Data Type Conversion76/1 -> Bus Assignment17/11
  Constant224/1 -> Bus Assignment14/10
  Constant135/1 -> Bus Assignment10/20
  Constant215/1 -> Data Type Conversion55/1
  Constant120/1 -> Data Type Conversion81/1
  Constant233/1 -> Bus Assignment14/19
  Constant138/1 -> Bus Assignment10/23
  Constant276/1 -> Data Type Conversion79/1
  Constant268/1 -> Bus Assignment16/6
  Constant169/1 -> Data Type Conversion35/1
  Constant147/1 -> Bus Assignment11/9
  Constant274/1 -> Bus Assignment16/10
  Constant293/1 -> Bus Assignment17/6
  Constant242/1 -> Data Type Conversion47/1
  Data Type Conversion33/1 -> Bus Assignment10/4
  Data Type Conversion62/1 -> Bus Assignment10/17
  Constant255/1 -> Bus Assignment15/16
  Constant211/1 -> Bus Assignment13/22
  Constant298/1 -> Bus Assignment17/8
  Constant204/1 -> Bus Assignment13/14
  Constant206/1 -> Bus Assignment13/18
  Data Type Conversion80/1 -> Bus Assignment16/5
  Constant304/1 -> Bus Assignment17/14
  Constant213/1 -> Bus Assignment13/23
  Data Type Conversion81/1 -> Bus Assignment10/5
  Data Type Conversion37/1 -> Bus Assignment14/4
  Constant214/1 -> Bus Assignment13/25
  Constant290/1 -> Data Type Conversion77/1
  Data Type Conversion36/1 -> Bus Assignment13/4
  Constant251/1 -> Data Type Conversion68/1
  Constant217/1 -> Data Type Conversion46/1
  Constant117/1 -> Data Type Conversion43/1
  Constant130/1 -> Bus Assignment10/16
  Constant212/1 -> Bus Assignment13/24
  Constant267/1 -> Data Type Conversion52/1
  Constant291/1 -> Bus Assignment17/2
  Constant307/1 -> Data Type Conversion74/1
  Constant183/1 -> Bus Assignment12/19
  Constant146/1 -> Bus Assignment11/7
  Constant174/1 -> Bus Assignment12/10
  Data Type Conversion48/1 -> Bus Assignment13/3
  Data Type Conversion69/1 -> Bus Assignment14/26
  Constant201/1 -> Data Type Conversion65/1
  Constant231/1 -> Bus Assignment14/18
  Constant207/1 -> Data Type Conversion56/1
  Data Type Conversion46/1 -> Bus Assignment14/3
  Constant208/1 -> Bus Assignment13/19
  Constant168/1 -> Bus Assignment12/6
  Constant262/1 -> Bus Assignment15/24
  Constant272/1 -> Bus Assignment16/9
  Bus Assignment10/1 -> Matrix Concatenate1/7
  Matrix Concatenate1/1 -> Bus Assignment9/4
  Data Type Conversion87/1 -> Bus Assignment9/7
  Data Type Conversion88/1 -> Bus Assignment9/8
  Data Type Conversion89/1 -> Bus Assignment9/9
  Blank Message19/1 -> Bus Assignment19/1
  Constant341/1 -> Bus Assignment19/2
  Bus Assignment19/1 -> Publish7/1
  Constant342/1 -> Data Type Conversion90/1
  Data Type Conversion90/1 -> Bus Assignment19/3
  Blank Message20/1 -> Bus Assignment20/1
  String Constant5/1(Out1) -> String Length5/1(In1), String to ASCII5/1(In1)
  String to ASCII5/1(Out1) -> Bus Assignment20/2
  String Length5/1(Out1) -> Bus Assignment20/3
  Constant343/1 -> Bus Assignment20/4
  Constant344/1 -> Bus Assignment20/5
  Constant345/1 -> Bus Assignment20/6
  String Length6/1(Out1) -> Bus Assignment21/3
  Blank Message21/1 -> Bus Assignment21/1
  Constant348/1 -> Bus Assignment21/6
  String Constant6/1(Out1) -> String Length6/1(In1), String to ASCII6/1(In1)
  Constant346/1 -> Bus Assignment21/4
  Constant347/1 -> Bus Assignment21/5
  String to ASCII6/1(Out1) -> Bus Assignment21/2
  Bus Assignment20/1 -> Matrix Concatenate2/1
  Bus Assignment21/1 -> Matrix Concatenate2/2
  Matrix Concatenate2/1 -> Bus Assignment19/4
  Data Type Conversion99/1 -> Bus Assignment23/15
  Constant359/1 -> Data Type Conversion99/1
  Constant354/1 -> Bus Assignment23/10
  Data Type Conversion92/1 -> Bus Assignment22/3
  Bus Assignment26/1 -> Bus Assignment23/9
  Data Type Conversion98/1 -> Bus Assignment23/11
  Data Type Conversion96/1 -> Bus Assignment23/14
  Constant360/1 -> Data Type Conversion92/1
  Data Type Conversion97/1 -> Bus Assignment27/5
  Constant351/1 -> Data Type Conversion94/1
  Constant350/1 -> Bus Assignment26/4, Bus Assignment26/3, Bus Assignment26/2
  Constant357/1 -> Data Type Conversion96/1
  Constant364/1 -> Bus Assignment24/2, Bus Assignment24/4, Bus Assignment24/3
  Blank Message23/1 -> Bus Assignment23/1
  Constant352/1 -> Data Type Conversion95/1
  Constant353/1 -> Bus Assignment23/13
  Constant358/1 -> Data Type Conversion97/1
  Bus Assignment24/1 -> Bus Assignment23/3
  Constant355/1 -> Data Type Conversion98/1
  Data Type Conversion95/1 -> Bus Assignment27/4
  Blank Message24/1 -> Bus Assignment26/1, Bus Assignment25/1, Bus Assignment24/1
  Data Type Conversion91/1 -> Bus Assignment22/2
  Bus Assignment25/1 -> Bus Assignment23/5
  Constant356/1 -> Bus Assignment23/12
  Constant349/1 -> Data Type Conversion91/1
  Constant367/1 -> Bus Assignment23/8
  Bus Assignment27/1 -> Publish8/1
  Bus Assignment22/1 -> Bus Assignment27/3
  Constant361/1 -> Data Type Conversion93/1
  Constant365/1 -> Bus Assignment23/6
  Blank Message22/1 -> Bus Assignment22/1
  Constant363/1 -> Bus Assignment23/4
  Data Type Conversion93/1 -> Bus Assignment22/6, Bus Assignment22/4, Bus Assignment22/5
  Constant362/1 -> Bus Assignment25/4, Bus Assignment25/3, Bus Assignment25/2
  Data Type Conversion94/1 -> Bus Assignment23/2
  Bus Assignment23/1 -> Bus Assignment27/2
  Blank Message25/1 -> Bus Assignment27/1
  Constant366/1 -> Bus Assignment23/7

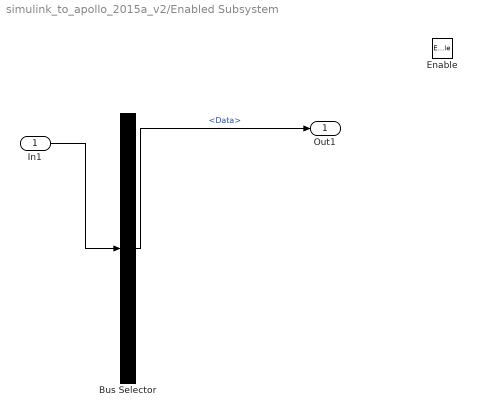
== system simulink_to_apollo_2015a_v2/Enabled Subsystem ==
  In1 : Inport
  Enable : EnablePort
  Bus Selector : BusSelector  DialogController=Simulink.DDGSource_BusSelector  OutputSignals=Data
  Out1 : Outport
  wires:
  In1/1 -> Bus Selector/1
  Bus Selector/1 -> Out1/1  "<Data>"

== system simulink_to_apollo_2015a_v2/String Constant1 ==
  Ground1 : Ground
  Out1 : Outport
  wires:
  Ground1/1 -> Out1/1

== system simulink_to_apollo_2015a_v2/String Constant2 ==
  Ground1 : Ground
  Out1 : Outport
  wires:
  Ground1/1 -> Out1/1

== system simulink_to_apollo_2015a_v2/String Constant3 ==
  Ground1 : Ground
  Out1 : Outport
  wires:
  Ground1/1 -> Out1/1

== system simulink_to_apollo_2015a_v2/String Constant4 ==
  Ground1 : Ground
  Out1 : Outport
  wires:
  Ground1/1 -> Out1/1

== system simulink_to_apollo_2015a_v2/String Constant5 ==
  Ground1 : Ground
  Out1 : Outport
  wires:
  Ground1/1 -> Out1/1

== system simulink_to_apollo_2015a_v2/String Constant6 ==
  Ground1 : Ground
  Out1 : Outport
  wires:
  Ground1/1 -> Out1/1

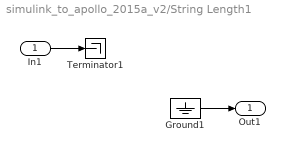
== system simulink_to_apollo_2015a_v2/String Length1 ==
  In1 : Inport
  Ground1 : Ground
  Terminator1 : Terminator
  Out1 : Outport
  wires:
  Ground1/1 -> Out1/1
  In1/1 -> Terminator1/1

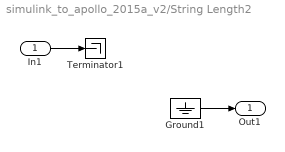
== system simulink_to_apollo_2015a_v2/String Length2 ==
  In1 : Inport
  Ground1 : Ground
  Terminator1 : Terminator
  Out1 : Outport
  wires:
  Ground1/1 -> Out1/1
  In1/1 -> Terminator1/1

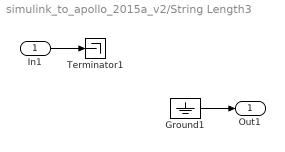
== system simulink_to_apollo_2015a_v2/String Length3 ==
  In1 : Inport
  Ground1 : Ground
  Terminator1 : Terminator
  Out1 : Outport
  wires:
  Ground1/1 -> Out1/1
  In1/1 -> Terminator1/1

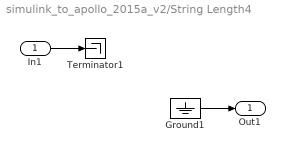
== system simulink_to_apollo_2015a_v2/String Length4 ==
  In1 : Inport
  Ground1 : Ground
  Terminator1 : Terminator
  Out1 : Outport
  wires:
  Ground1/1 -> Out1/1
  In1/1 -> Terminator1/1

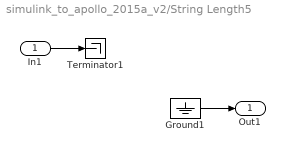
== system simulink_to_apollo_2015a_v2/String Length5 ==
  In1 : Inport
  Ground1 : Ground
  Terminator1 : Terminator
  Out1 : Outport
  wires:
  Ground1/1 -> Out1/1
  In1/1 -> Terminator1/1

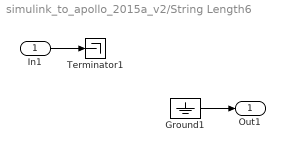
== system simulink_to_apollo_2015a_v2/String Length6 ==
  In1 : Inport
  Ground1 : Ground
  Terminator1 : Terminator
  Out1 : Outport
  wires:
  Ground1/1 -> Out1/1
  In1/1 -> Terminator1/1

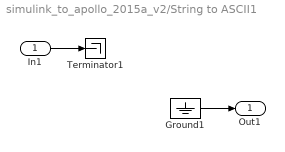
== system simulink_to_apollo_2015a_v2/String to ASCII1 ==
  In1 : Inport
  Ground1 : Ground
  Terminator1 : Terminator
  Out1 : Outport
  wires:
  Ground1/1 -> Out1/1
  In1/1 -> Terminator1/1

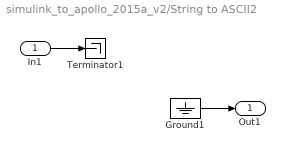
== system simulink_to_apollo_2015a_v2/String to ASCII2 ==
  In1 : Inport
  Ground1 : Ground
  Terminator1 : Terminator
  Out1 : Outport
  wires:
  Ground1/1 -> Out1/1
  In1/1 -> Terminator1/1

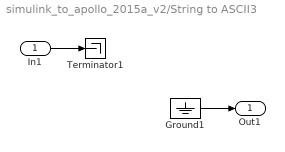
== system simulink_to_apollo_2015a_v2/String to ASCII3 ==
  In1 : Inport
  Ground1 : Ground
  Terminator1 : Terminator
  Out1 : Outport
  wires:
  Ground1/1 -> Out1/1
  In1/1 -> Terminator1/1

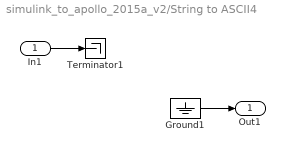
== system simulink_to_apollo_2015a_v2/String to ASCII4 ==
  In1 : Inport
  Ground1 : Ground
  Terminator1 : Terminator
  Out1 : Outport
  wires:
  Ground1/1 -> Out1/1
  In1/1 -> Terminator1/1

== system simulink_to_apollo_2015a_v2/String to ASCII5 ==
  In1 : Inport
  Ground1 : Ground
  Terminator1 : Terminator
  Out1 : Outport
  wires:
  Ground1/1 -> Out1/1
  In1/1 -> Terminator1/1

== system simulink_to_apollo_2015a_v2/String to ASCII6 ==
  In1 : Inport
  Ground1 : Ground
  Terminator1 : Terminator
  Out1 : Outport
  wires:
  Ground1/1 -> Out1/1
  In1/1 -> Terminator1/1
